simulink model "system_model_2021_sym"  (R2021b)
settings: Solver=FixedStepAuto  StartTime=0.0  StopTime=10  RelTol=1e-3
values from neighbouring files (symbols this model uses):
  init_theta_1 = pi    (= 3.14159265359)    [Copy_of_step2_whitebox_beam.m]    (also in compare_ourmodel_with_others.m = 0; linearize_script.m; step2_whitebox_beam.m; syms_test.m)
  init_theta_2 = -pi/2    (= -1.57079632679)    [Copy_of_step2_whitebox_beam.m]    (also in compare_ourmodel_with_others.m = 0; linearize_script.m = 1.57079632679; step2_whitebox_beam.m; syms_test.m = 0)
settings Model: Creator=97083  LastModifiedBy=lyitingli
settings DataIOCC: ExternalInput=[u]
settings DebuggingCC: UnconnectedInputMsg=none  UnconnectedOutputMsg=none  UnconnectedLineMsg=none  UnderSpecifiedDimensionMsg=warning
settings ModelReferenceCC: EnableRefExpFcnMdlSchedulingChecks=off
settings RTWCC: DLArmComputeVersion=20.02.1

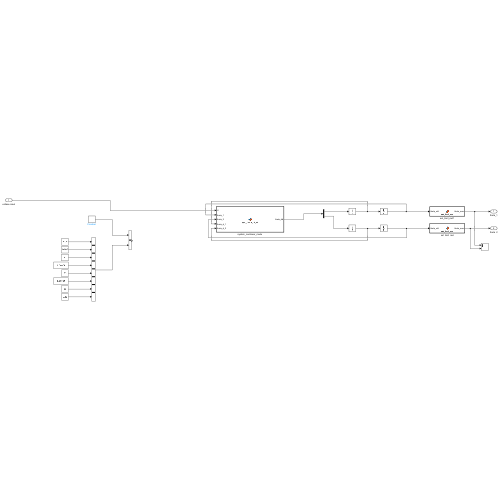
[thumbnail: Simulink's stored preview of the top-level diagram]
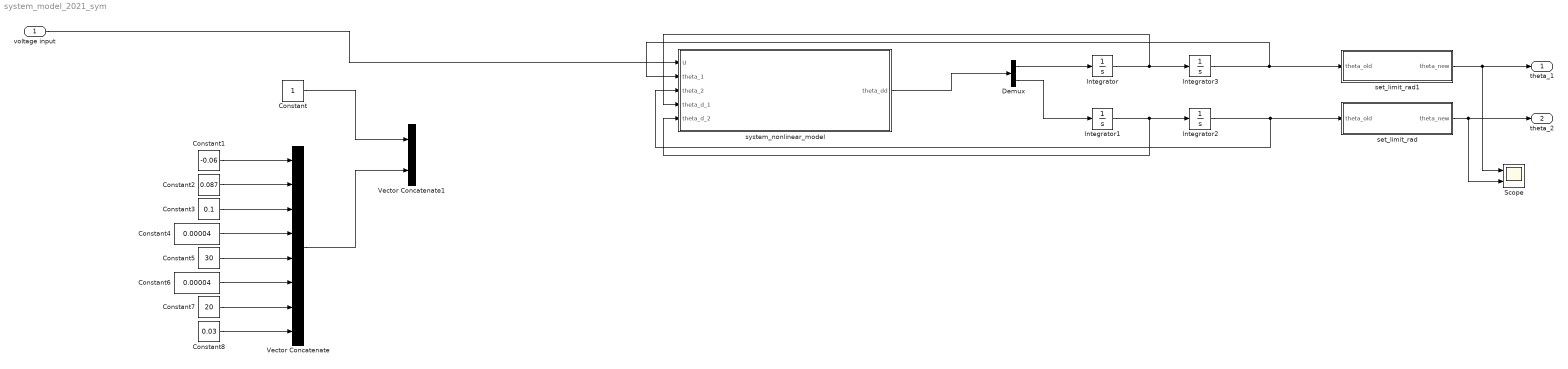
== system system_model_2021_sym ==
  voltage input : Inport  LockScale=on
  Constant : Constant
  Constant1 : Constant  Value=-0.06
  Constant2 : Constant  Value=0.087
  Constant3 : Constant  Value=0.1
  Constant4 : Constant  Value=0.00004
  Constant5 : Constant  Value=30
  Constant6 : Constant  Value=0.00004
  Constant7 : Constant  Value=20
  Constant8 : Constant  Value=0.03
  Demux : Demux  Outputs=2
  Integrator : Integrator
  Integrator1 : Integrator
  Integrator2 : Integrator  InitialCondition=init_theta_2
  Integrator3 : Integrator  InitialCondition=init_theta_1
  Scope : Scope  NumInputPorts=2
  Vector Concatenate : Concatenate  NumInputs=8
  Vector Concatenate1 : Concatenate
  set_limit_rad : MATLAB Function  TreatAsAtomicUnit=on
  set_limit_rad1 : MATLAB Function  TreatAsAtomicUnit=on
  system_nonlinear_model : MATLAB Function  TreatAsAtomicUnit=on
  theta_1 : Outport
  theta_2 : Outport  Port=2
  wires:
  system_nonlinear_model/1(theta_dd) -> Demux/1
  Demux/1 -> Integrator/1
  Integrator/1 -> system_nonlinear_model/4(theta_d_1), Integrator3/1
  Demux/2 -> Integrator1/1
  Integrator1/1 -> system_nonlinear_model/5(theta_d_2), Integrator2/1
  Integrator3/1 -> set_limit_rad1/1(theta_old), system_nonlinear_model/2(theta_1)
  Integrator2/1 -> system_nonlinear_model/3(theta_2), set_limit_rad/1(theta_old)
  set_limit_rad/1(theta_new) -> Scope/2, theta_2/1
  set_limit_rad1/1(theta_new) -> Scope/1, theta_1/1
  Constant1/1 -> Vector Concatenate/1
  Constant2/1 -> Vector Concatenate/2
  Constant3/1 -> Vector Concatenate/3
  Constant4/1 -> Vector Concatenate/4
  Constant5/1 -> Vector Concatenate/5
  Constant6/1 -> Vector Concatenate/6
  Constant7/1 -> Vector Concatenate/7
  Constant8/1 -> Vector Concatenate/8
  Constant/1 -> Vector Concatenate1/1
  Vector Concatenate/1 -> Vector Concatenate1/2
  voltage input/1 -> system_nonlinear_model/1(U)

== matlab function system_model_2021_sym/set_limit_rad ==
  settings: updateMethod=DISCRETE  sampleTime=0.001
  data: theta_old input size=1; theta_new output size=1
function theta_new   = set_limit_rad(theta_old)

theta_new = theta_old - floor((theta_old + 0.5*pi) / 2 / pi) * 2 * pi;

theta_new = theta_old;

== matlab function system_model_2021_sym/system_nonlinear_model ==
  settings: updateMethod=DISCRETE  sampleTime=0.001
  data: U input size=9; theta_dd output size=2; theta_1 input size=1; theta_2 input size=1; theta_d_1 input size=1; theta_d_2 input size=1
function theta_dd   = get_theta_dt_dt(U, theta_1, theta_2, theta_d_1, theta_d_2)

% constant variables
g = 9.81;
l_1 = 0.1;
l_2 = 0.1;
m_1 = 0.125;
m_2 = 0.05;
% params = [-0.04, 0.06, 0.074, 0.00002, 4.8, 0.00077, 50, 0.03];


% varying variables
u = U(1);
c_1_0 = U(2);
c_2_0 = U(3);
I_1_0 = U(4);
I_2_0 = U(5);
b_1_0 = U(6);
b_2_0 = U(7);
k_m_0 = U(8);
tau_e_0 = U(9);


% calculate other variables
P_1 = m_1 * c_1_0 * c_1_0 + m_2 * l_1 * l_1 + I_1_0;
P_2 = m_2 * c_2_0 * c_2_0 + I_2_0;
P_3 = m_2 * l_1 * c_2_0;

g_1 = (m_1 * c_1_0 + m_2 * l_1) * g;
g_2 = m_2 * c_2_0 * g;


% construct the vector for matrix calculation

% theta_vec = [theta_1; theta_2];
theta_d_vec = [theta_d_1; theta_d_2];
% theta_d_d_vec = [theta_1; theta_2];
T = k_m_0 * u;
T_vec = [T; 0];
theta_dd = zeros(2, 1);

% matrix
M = [P_1 + P_2 + 2 * P_3 * cos(theta_2) P_2 + P_3 * cos(theta_2);
    P_2 + P_3 * cos(theta_2)            P_2];

C = [b_1_0 - P_3 * theta_d_2 * sin(theta_2)  -P_3 * (theta_d_1 + theta_d_2) * sin(theta_2);
    P_3 * theta_d_1 * sin(theta_2)           b_2_0];

G = [-g_1 * sin(theta_1) - g_2 * sin(theta_1 + theta_2);
     -g_2 * sin(theta_1 + theta_2)];

M_inv = inv(M);

theta_dd = M_inv * T_vec - M_inv * C * theta_d_vec- M_inv * G;

== matlab function system_model_2021_sym/set_limit_rad1 ==
  settings: updateMethod=DISCRETE  sampleTime=0.001
  data: theta_old input size=1; theta_new output size=1
function theta_new   = set_limit_rad(theta_old)

theta_new = theta_old - floor((theta_old + 0.5*pi) / 2 / pi) * 2 * pi;
theta_new = theta_old;
